simulink model "modelo3"  (R2019a)
settings: Solver=FixedStepAuto  StartTime=0.0  StopTime=tfinal  FixedStep=0.0001  RelTol=1e-3
values from neighbouring files (symbols this model uses):
  A = 4*10^(-4)    (= 0.0004)    [nonlinear.m]    (also in sim2.m = [zeros(2) eye(2);Ke*eye(2) -Ge]; sim3.m = [zeros(2) eye(2);Ke*eye(2) -Ge]; sim4.m = [zeros(2) eye(2);Ke*eye(2) -Ge])
  B = (1/J)*d*b*ki*[zeros(2);eye(2)]    [sim2.m]    (also in sim3.m = (1/J)*d*b*gi*[zeros(2);eye(2)]; sim4.m = (1/J)*d*b*gi*[zeros(2);eye(2)])
  C = [eye(2) zeros(2)]    [sim2.m]    (also in sim3.m; sim4.m)
  D = zeros(2)    [sim2.m]    (also in sim3.m = zeros(4,2); sim4.m = zeros(4,2))
  F = lqr(A,B,Q,R)    [descentralizado.m]    (also in sim2.m = Fdn)
  M = 0.5    [sim3.m]    (also in sim4.m)
  omega = 4000    [sim2.m]    (also in sim3.m = 356; sim4.m = 3204)
  x0 = [0.0002;-0.0002;0;0]    [sim2.m]    (also in sim3.m; sim4.m)
settings Model: Creator=vinic  LastModifiedBy=vinic
settings DataIOCC: ReturnWorkspaceOutputs=off
settings DebuggingCC: PregeneratedLibrarySubsystemCodeDiagnostic=none  ArithmeticOperatorsInVariantConditions=warning
settings SFSimCC: SimUseLocalCustomCode=off
settings RTWCC: RTWUseLocalCustomCode=off

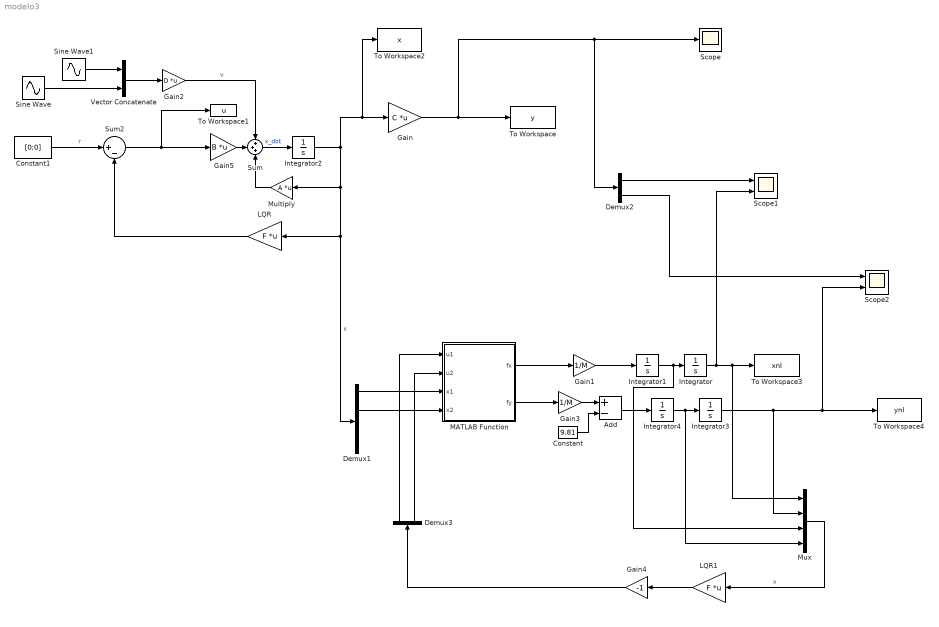
== system modelo3 ==
  Add : Sum  Inputs=+-
  Constant : Constant  Value=9.81
  Constant1 : Constant  Value=[0;0]  VectorParams1D=off
  Demux1 : Demux
  Demux2 : Demux  Outputs=2
  Demux3 : Demux  Outputs=2
  Gain : Gain  Gain=C  Multiplication=Matrix(K*u)
  Gain1 : Gain  Gain=1/M
  Gain2 : Gain  Gain=D  Multiplication=Matrix(K*u)
  Gain3 : Gain  Gain=1/M
  Gain4 : Gain  Gain=-1
  Gain5 : Gain  Gain=B  Multiplication=Matrix(K*u)
  Integrator : Integrator  InitialCondition=x0(1)
  Integrator1 : Integrator  InitialCondition=x0(1)
  Integrator2 : Integrator  InitialCondition=x0
  Integrator3 : Integrator  InitialCondition=x0(2)
  Integrator4 : Integrator  InitialCondition=x0(2)
  LQR : Gain  Gain=F  Multiplication=Matrix(K*u)
  LQR1 : Gain  Gain=F  Multiplication=Matrix(K*u)
  MATLAB Function : MATLAB Function  TreatAsAtomicUnit=on
  Multiply : Gain  Gain=A  Multiplication=Matrix(K*u)
  Mux : Mux
  Scope : Scope
  Scope1 : Scope  NumInputPorts=2
  Scope2 : Scope  NumInputPorts=2
  Sine Wave : Sin  Amplitude=-1  Frequency=omega  SampleTime=0
  Sine Wave1 : Sin  Frequency=omega  Phase=-pi/2  SampleTime=0
  Sum : Sum  Inputs=+++
  Sum2 : Sum  Inputs=|+-
  To Workspace : ToWorkspace  VariableName=y  SampleTime=-1
  To Workspace1 : ToWorkspace  VariableName=u  SampleTime=-1
  To Workspace2 : ToWorkspace  VariableName=x  SampleTime=-1
  To Workspace3 : ToWorkspace  VariableName=xnl  SampleTime=-1
  To Workspace4 : ToWorkspace  VariableName=ynl  SampleTime=-1
  Vector Concatenate : Concatenate
  wires:
  Sum2/1 -> To Workspace1/1, Gain5/1
  Integrator2/1 -> Demux1/1, LQR/1, Multiply/1, To Workspace2/1, Gain/1  "x"
  Gain/1 -> Demux2/1, Scope/1, To Workspace/1
  Gain5/1 -> Sum/2
  Multiply/1 -> Sum/3
  Sum/1 -> Integrator2/1  "x_dot"
  Gain2/1 -> Sum/1  "v"
  LQR/1 -> Sum2/2
  Sine Wave1/1 -> Vector Concatenate/1
  Sine Wave/1 -> Vector Concatenate/2
  Vector Concatenate/1 -> Gain2/1
  Constant1/1 -> Sum2/1  "r"
  Constant/1 -> Add/2
  Gain3/1 -> Add/1
  Demux1/1 -> MATLAB Function/3(x1)
  Demux1/2 -> MATLAB Function/4(x2)
  MATLAB Function/1(fx) -> Gain1/1
  MATLAB Function/2(fy) -> Gain3/1
  Gain1/1 -> Integrator1/1
  Integrator1/1 -> Mux/3, Integrator/1
  Integrator/1 -> Mux/1, To Workspace3/1, Scope1/2
  Add/1 -> Integrator4/1
  Integrator4/1 -> Mux/4, Integrator3/1
  Integrator3/1 -> Mux/2, Scope2/2, To Workspace4/1
  Demux2/1 -> Scope1/1
  Demux2/2 -> Scope2/1
  Mux/1 -> LQR1/1  "x"
  LQR1/1 -> Gain4/1
  Gain4/1 -> Demux3/1
  Demux3/1 -> MATLAB Function/1(u1)
  Demux3/2 -> MATLAB Function/2(u2)

== matlab function modelo3/MATLAB Function ==
  data: u1 input; u2 input; fx output; x1 input; x2 input; fy output
function [fx,fy] = nonlinearMB(u1,   u2,   x1,   x2)

mu = 4*pi*10^(-7); %permeabilidade mag. do vácuo
A = 4*10^(-4); %área superficial do polo
h = 0.5*10^(-3); %entreferro
n = 300; %número de espiras da bobina
i0 = 0.2325; %corrente de base, na dissertação é iB1
g = 9.81;


id3 = (3/sqrt(3))*u1;
id1 = u2;

N1 = 6*(i0)^2*h*x1 + 3*(i0)^2*x1*x2 + 4*sqrt(3)*(i0)*h^2*(id3) + 12*i0*h*(id1)*x1 + 6*i0*(id1)*x1*x2 + sqrt(3)*(i0)*(id3)*x1^2 -sqrt(3)*(i0)*(id3)*x2^2 + 4*sqrt(3)*h^2*(id1)*(id3) + 6*h*(id1)^2*x1 + 2*h*(id3)^2*x1 + 3*(id1)^2*x1*x2 + sqrt(3)*(id1)*(id3)*x1^2 - sqrt(3)*(id1)*(id3)*x2^2 - (id3)^2*x1*x2;

N2 = 12*(i0)^2*h^2 + 12*(i0)^2*h*x2 - 3*(i0)^2*x1^2 + 3*(i0)^2*x2^2 + 24*(i0)*h^2*(id1) + 24*(i0)*h*x2*(id1) - 6*(i0)*(id1)*x1^2 + 6*(i0)*(id1)*x2^2 + 4*sqrt(3)*i0*(id3)*x1*x2 + 12*h^2*(id1)^2 - 4*h^2*(id3)^2 + 12*h*(id1)^2*x2 + 4*h*(id3)^2*x2 - 3*(id1)^2*x1^2 + 3*(id1)^2*x2^2 + 4*sqrt(3)*(id1)*(id3)*x1*x2 + (id3)^2*x1^2 -(id3)^2*x2^2;

DELTA = (x1^2 + x2^2 - 4*h^2);

fx = (4/3)*mu*A*n^2*N1/DELTA^2;
fy = (2/3)*mu*A*n^2*N2/DELTA^2;

%https://blogs.mathworks.com/loren/2013/06/10/from-symbolic-differential-equations-to-their-numeric-solution/
%solução simbólica
% ode1 = diff(x,2) == (1/m)*fx;
% ode2 = diff(y,2) == -g + (1/m)*fy;
% 
% V = odeToVectorField(ode1,ode2);
% 
% F = matlabFunction(V,'vars',{'t','x','y'})
% 
% sol = ode45(F,t,2*10^(-4) -2*10^(-4));

% ynl = zeros(4,1);
% ynl(1) = x(3);
% ynl(2) = x(4);
% ynl(3) =(1/m)*fx;
% ynl(4) = -g + (1/m)*fy;

%ynl = ode45()

end
